simulink model "MyInverter_RTW"  (R2022a)
settings: Solver=ode1  StartTime=0.0  StopTime=inf  FixedStep=0.0002  RelTol=1e-3
PreLoadFcn:
  | vehicle = 'Car'; if ~length(which('cmself')), cmenv; end
  | MyInverter_RTW_bus
InitFcn:
  | vehicle = 'Car'; if ~length(which('cmself')), cmenv; end
  | MyInverter_RTW_bus
Description:
  | CarMaker Plug-in Model Target
settings Model: Creator=ml  LastModifiedBy=IPG
settings DebuggingCC: UnconnectedInputMsg=warning  UnconnectedOutputMsg=warning  UnconnectedLineMsg=warning
settings RTWCC: Description=CarMaker Plug-in Model Target  SystemTargetFile=CarMaker.tlc  TemplateMakefile=CarMaker_unix-win64.tmf  DLArmComputeVersion=19.05
settings CodeAppCC: MaxIdLength=127
settings STFCustomTargetCC: TargetLangStandard=C99 (ISO)  CombineOutputUpdateFcns=on  MatFileLogging=on  CodeInterfacePackaging=Reusable function  GRTInterface=off  GenerateAllocFcn=on  SystemTargetFile=CarMaker.tlc
settings GRTTargetCC: ParMdlRefBuildCompliant=off  CompOptLevelCompliant=off  ConcurrentExecutionCompliant=off  CodeInterfacePackaging=Reusable function  CPPClassGenCompliant=off  GenerateAllocFcn=on  UseToolchainInfoCompliant=off

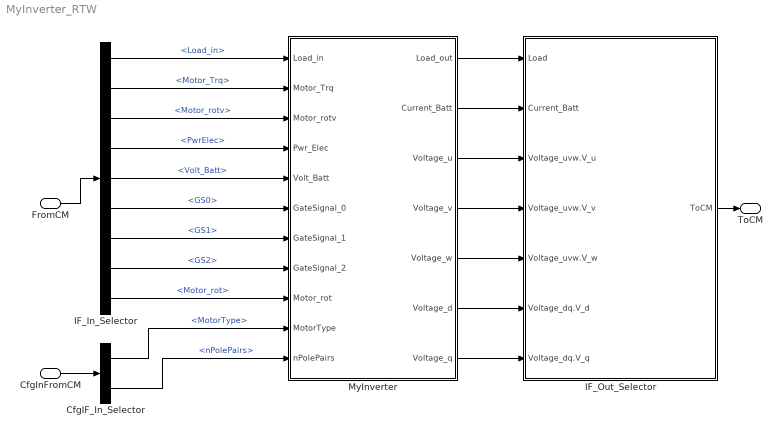
== system MyInverter_RTW ==
  FromCM : Inport  OutDataTypeStr=Bus: cmPTInverterIn
  CfgInFromCM : Inport  Port=2  OutDataTypeStr=Bus: cmPTInverterCfgIn
  CfgIF_In_Selector : BusSelector  OutputSignals=MotorType,nPolePairs
  IF_In_Selector : BusSelector  OutputSignals=Load_in,Motor_Trq,Motor_rotv,PwrElec,Volt_Batt,GateSignal.GS0,GateSignal.GS1,GateSignal.GS2,Motor_rot
  IF_Out_Selector : Subsystem  mask(Signal Selection){}
      mask help: Signal Selection Block
      settings: OpenFcn=cmSignalSelect('SignalSelection_CB',gcb)
  MyInverter : Subsystem
  ToCM : Outport  OutDataTypeStr=Bus: cmPTInverterOut
  wires:
  FromCM/1 -> IF_In_Selector/1
  IF_Out_Selector/1(ToCM) -> ToCM/1
  CfgInFromCM/1 -> CfgIF_In_Selector/1
  MyInverter/6(Voltage_d) -> IF_Out_Selector/6(Voltage_dq.V_d)
  IF_In_Selector/4 -> MyInverter/4(Pwr_Elec)  "<PwrElec>"
  IF_In_Selector/6 -> MyInverter/6(GateSignal_0)  "<GS0>"
  MyInverter/1(Load_out) -> IF_Out_Selector/1(Load)
  IF_In_Selector/9 -> MyInverter/9(Motor_rot)  "<Motor_rot>"
  IF_In_Selector/3 -> MyInverter/3(Motor_rotv)  "<Motor_rotv>"
  IF_In_Selector/2 -> MyInverter/2(Motor_Trq)  "<Motor_Trq>"
  MyInverter/5(Voltage_w) -> IF_Out_Selector/5(Voltage_uvw.V_w)
  CfgIF_In_Selector/2 -> MyInverter/11(nPolePairs)  "<nPolePairs>"
  IF_In_Selector/1 -> MyInverter/1(Load_in)  "<Load_in>"
  IF_In_Selector/7 -> MyInverter/7(GateSignal_1)  "<GS1>"
  MyInverter/3(Voltage_u) -> IF_Out_Selector/3(Voltage_uvw.V_u)
  IF_In_Selector/8 -> MyInverter/8(GateSignal_2)  "<GS2>"
  MyInverter/4(Voltage_v) -> IF_Out_Selector/4(Voltage_uvw.V_v)
  MyInverter/2(Current_Batt) -> IF_Out_Selector/2(Current_Batt)
  IF_In_Selector/5 -> MyInverter/5(Volt_Batt)  "<Volt_Batt>"
  MyInverter/7(Voltage_q) -> IF_Out_Selector/7(Voltage_dq.V_q)
  CfgIF_In_Selector/1 -> MyInverter/10(MotorType)  "<MotorType>"

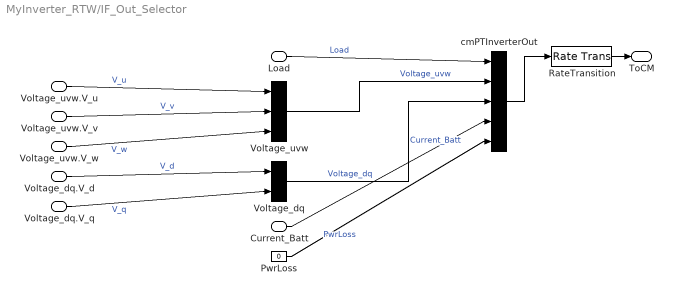
== system MyInverter_RTW/IF_Out_Selector ==
  Load : Inport
  Current_Batt : Inport  Port=2
  Voltage_uvw.V_u : Inport  Port=3
  Voltage_uvw.V_v : Inport  Port=4
  Voltage_uvw.V_w : Inport  Port=5
  Voltage_dq.V_d : Inport  Port=6
  Voltage_dq.V_q : Inport  Port=7
  PwrLoss : Constant  Value=0
  RateTransition : RateTransition  OutPortSampleTime=str2num(get_param(bdroot,'FixedStep'))
  Voltage_dq : BusCreator  Inputs=2
  Voltage_uvw : BusCreator  Inputs=3
  cmPTInverterOut : BusCreator  Inputs=5
  ToCM : Outport
  wires:
  RateTransition/1 -> ToCM/1
  cmPTInverterOut/1 -> RateTransition/1
  Voltage_uvw/1 -> cmPTInverterOut/2  "Voltage_uvw"
  Voltage_dq/1 -> cmPTInverterOut/3  "Voltage_dq"
  PwrLoss/1 -> cmPTInverterOut/5  "PwrLoss"
  Load/1 -> cmPTInverterOut/1  "Load"
  Current_Batt/1 -> cmPTInverterOut/4  "Current_Batt"
  Voltage_uvw.V_u/1 -> Voltage_uvw/1  "V_u"
  Voltage_uvw.V_v/1 -> Voltage_uvw/2  "V_v"
  Voltage_uvw.V_w/1 -> Voltage_uvw/3  "V_w"
  Voltage_dq.V_d/1 -> Voltage_dq/1  "V_d"
  Voltage_dq.V_q/1 -> Voltage_dq/2  "V_q"

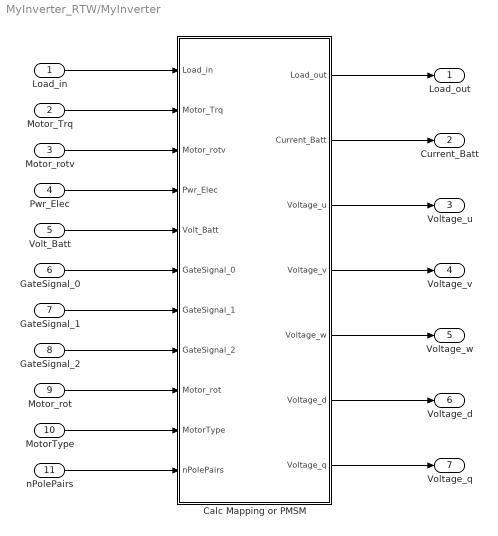
== system MyInverter_RTW/MyInverter ==
  Load_in : Inport
  Motor_Trq : Inport  Port=2
  Motor_rotv : Inport  Port=3
  Pwr_Elec : Inport  Port=4
  Volt_Batt : Inport  Port=5
  GateSignal_0 : Inport  Port=6
  GateSignal_1 : Inport  Port=7
  GateSignal_2 : Inport  Port=8
  Motor_rot : Inport  Port=9
  MotorType : Inport  Port=10
  nPolePairs : Inport  Port=11
  Calc Mapping or PMSM : Subsystem
  Load_out : Outport
  Current_Batt : Outport  Port=2
  Voltage_u : Outport  Port=3
  Voltage_v : Outport  Port=4
  Voltage_w : Outport  Port=5
  Voltage_d : Outport  Port=6
  Voltage_q : Outport  Port=7
  wires:
  Load_in/1 -> Calc Mapping or PMSM/1(Load_in)
  Motor_Trq/1 -> Calc Mapping or PMSM/2(Motor_Trq)
  Motor_rotv/1 -> Calc Mapping or PMSM/3(Motor_rotv)
  Pwr_Elec/1 -> Calc Mapping or PMSM/4(Pwr_Elec)
  Volt_Batt/1 -> Calc Mapping or PMSM/5(Volt_Batt)
  Calc Mapping or PMSM/1(Load_out) -> Load_out/1
  Calc Mapping or PMSM/2(Current_Batt) -> Current_Batt/1
  Calc Mapping or PMSM/3(Voltage_u) -> Voltage_u/1
  Calc Mapping or PMSM/4(Voltage_v) -> Voltage_v/1
  Calc Mapping or PMSM/5(Voltage_w) -> Voltage_w/1
  Calc Mapping or PMSM/6(Voltage_d) -> Voltage_d/1
  Calc Mapping or PMSM/7(Voltage_q) -> Voltage_q/1
  GateSignal_0/1 -> Calc Mapping or PMSM/6(GateSignal_0)
  GateSignal_1/1 -> Calc Mapping or PMSM/7(GateSignal_1)
  GateSignal_2/1 -> Calc Mapping or PMSM/8(GateSignal_2)
  MotorType/1 -> Calc Mapping or PMSM/10(MotorType)
  Motor_rot/1 -> Calc Mapping or PMSM/9(Motor_rot)
  nPolePairs/1 -> Calc Mapping or PMSM/11(nPolePairs)

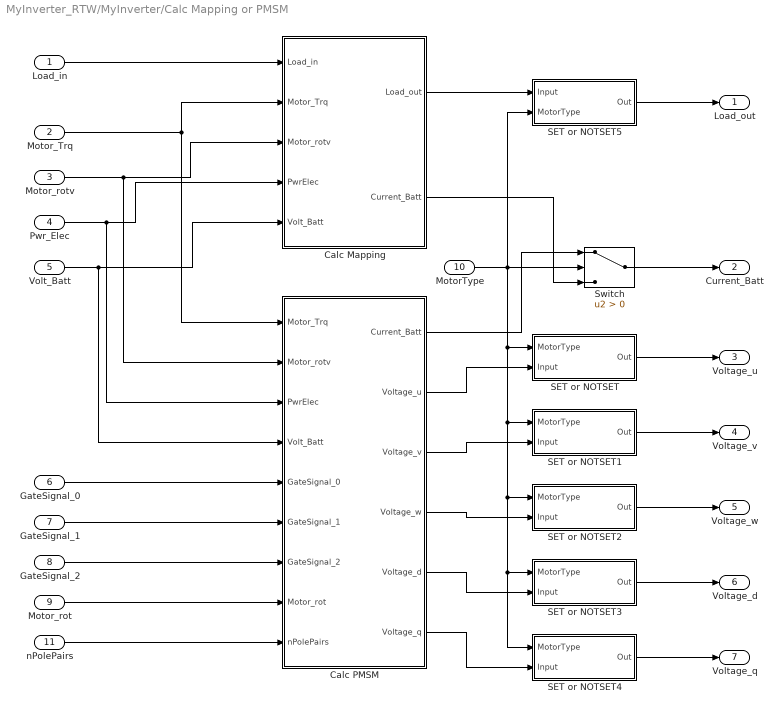
== system MyInverter_RTW/MyInverter/Calc Mapping or PMSM ==
  Load_in : Inport
  Motor_Trq : Inport  Port=2
  Motor_rotv : Inport  Port=3
  Pwr_Elec : Inport  Port=4
  Volt_Batt : Inport  Port=5
  GateSignal_0 : Inport  Port=6
  GateSignal_1 : Inport  Port=7
  GateSignal_2 : Inport  Port=8
  Motor_rot : Inport  Port=9
  MotorType : Inport  Port=10
  nPolePairs : Inport  Port=11
  Calc Mapping : Subsystem
  Calc PMSM : Subsystem
  SET or NOTSET : Subsystem
  SET or NOTSET1 : Subsystem
  SET or NOTSET2 : Subsystem
  SET or NOTSET3 : Subsystem
  SET or NOTSET4 : Subsystem
  SET or NOTSET5 : Subsystem
  Switch : Switch  Criteria=u2 > Threshold  SaturateOnIntegerOverflow=off  InputSameDT=off
  Load_out : Outport
  Current_Batt : Outport  Port=2
  Voltage_u : Outport  Port=3
  Voltage_v : Outport  Port=4
  Voltage_w : Outport  Port=5
  Voltage_d : Outport  Port=6
  Voltage_q : Outport  Port=7
  wires:
  Load_in/1 -> Calc Mapping/1(Load_in)
  Motor_Trq/1 -> Calc Mapping/2(Motor_Trq), Calc PMSM/1(Motor_Trq)
  Motor_rotv/1 -> Calc PMSM/2(Motor_rotv), Calc Mapping/3(Motor_rotv)
  Pwr_Elec/1 -> Calc PMSM/3(PwrElec), Calc Mapping/4(PwrElec)
  Volt_Batt/1 -> Calc PMSM/4(Volt_Batt), Calc Mapping/5(Volt_Batt)
  MotorType/1 -> SET or NOTSET5/2(MotorType), SET or NOTSET4/1(MotorType), SET or NOTSET3/1(MotorType), SET or NOTSET2/1(MotorType), SET or NOTSET1/1(MotorType), SET or NOTSET/1(MotorType), Switch/2
  Calc Mapping/2(Current_Batt) -> Switch/3
  Calc PMSM/1(Current_Batt) -> Switch/1
  Switch/1 -> Current_Batt/1
  Calc Mapping/1(Load_out) -> SET or NOTSET5/1(Input)
  GateSignal_0/1 -> Calc PMSM/5(GateSignal_0)
  GateSignal_1/1 -> Calc PMSM/6(GateSignal_1)
  GateSignal_2/1 -> Calc PMSM/7(GateSignal_2)
  Calc PMSM/2(Voltage_u) -> SET or NOTSET/2(Input)
  SET or NOTSET/1(Out) -> Voltage_u/1
  Calc PMSM/3(Voltage_v) -> SET or NOTSET1/2(Input)
  SET or NOTSET1/1(Out) -> Voltage_v/1
  Calc PMSM/4(Voltage_w) -> SET or NOTSET2/2(Input)
  SET or NOTSET2/1(Out) -> Voltage_w/1
  Calc PMSM/5(Voltage_d) -> SET or NOTSET3/2(Input)
  SET or NOTSET3/1(Out) -> Voltage_d/1
  Calc PMSM/6(Voltage_q) -> SET or NOTSET4/2(Input)
  SET or NOTSET4/1(Out) -> Voltage_q/1
  SET or NOTSET5/1(Out) -> Load_out/1
  Motor_rot/1 -> Calc PMSM/8(Motor_rot)
  nPolePairs/1 -> Calc PMSM/9(nPolePairs)

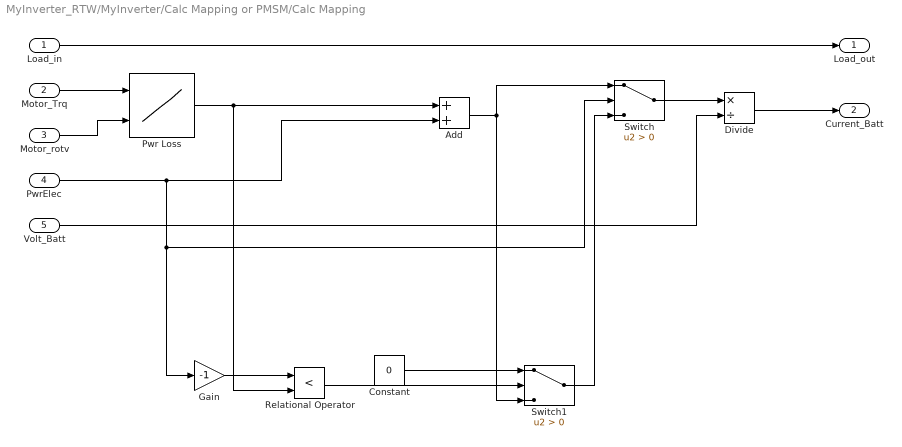
== system MyInverter_RTW/MyInverter/Calc Mapping or PMSM/Calc Mapping ==
  Load_in : Inport
  Motor_Trq : Inport  Port=2
  Motor_rotv : Inport  Port=3
  PwrElec : Inport  Port=4
  Volt_Batt : Inport  Port=5
  Add : Sum
  Constant : Constant  Value=0
  Divide : Product  Inputs=*/
  Gain : Gain  Gain=-1
  Pwr Loss : Lookup_n-D  BreakpointsForDimension1=[1,2,3]  BreakpointsForDimension2=[1,2,3]  Table=reshape([0,100,100,0,100,100,0,100,100],3,3)  InternalRulePriority=Speed  RndMeth=Simplest
      settings: InputPortMap=u0,u1
  Relational Operator : RelationalOperator  Operator=<  OutDataTypeStr=boolean  RndMeth=Simplest  InputSameDT=off
  Switch : Switch  Criteria=u2 > Threshold  SaturateOnIntegerOverflow=off  InputSameDT=off
  Switch1 : Switch  Criteria=u2 > Threshold  SaturateOnIntegerOverflow=off  InputSameDT=off
  Load_out : Outport
  Current_Batt : Outport  Port=2
  wires:
  Divide/1 -> Current_Batt/1
  Load_in/1 -> Load_out/1
  Switch1/1 -> Switch/3
  Gain/1 -> Relational Operator/1
  Motor_rotv/1 -> Pwr Loss/2
  Switch/1 -> Divide/1
  Pwr Loss/1 -> Relational Operator/2, Add/1
  Volt_Batt/1 -> Divide/2
  Motor_Trq/1 -> Pwr Loss/1
  Constant/1 -> Switch1/1
  Relational Operator/1 -> Switch1/2
  PwrElec/1 -> Gain/1, Switch/2, Add/2
  Add/1 -> Switch1/3, Switch/1

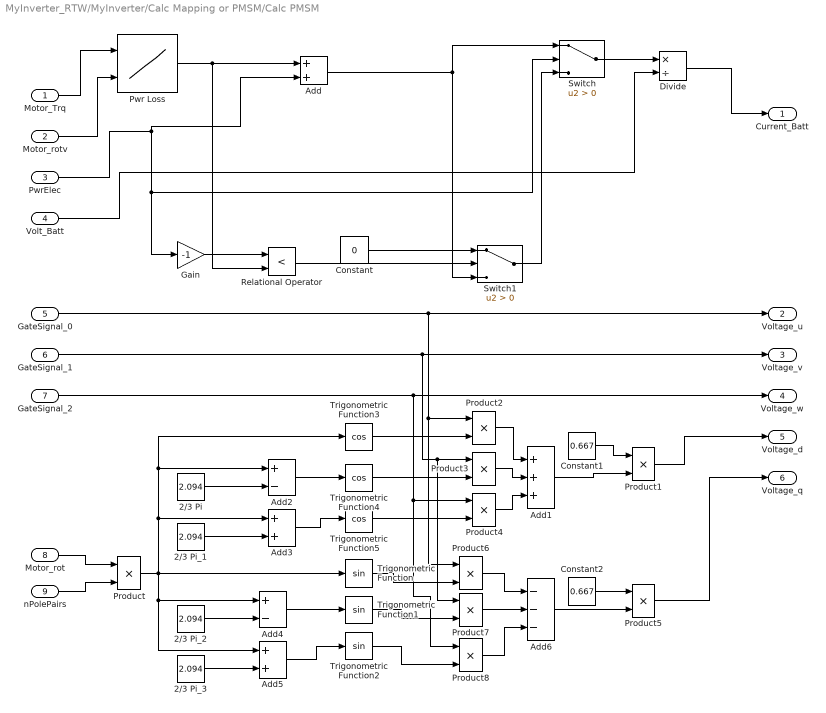
== system MyInverter_RTW/MyInverter/Calc Mapping or PMSM/Calc PMSM ==
  Motor_Trq : Inport
  Motor_rotv : Inport  Port=2
  PwrElec : Inport  Port=3
  Volt_Batt : Inport  Port=4
  GateSignal_0 : Inport  Port=5
  GateSignal_1 : Inport  Port=6
  GateSignal_2 : Inport  Port=7
  Motor_rot : Inport  Port=8
  nPolePairs : Inport  Port=9
  2/3 Pi : Constant  Value=2.094  OutDataTypeStr=double
  2/3 Pi_1 : Constant  Value=2.094  OutDataTypeStr=double
  2/3 Pi_2 : Constant  Value=2.094  OutDataTypeStr=double
  2/3 Pi_3 : Constant  Value=2.094  OutDataTypeStr=double
  Add : Sum
  Add1 : Sum  Inputs=+++
  Add2 : Sum  Inputs=+-
  Add3 : Sum
  Add4 : Sum  Inputs=+-
  Add5 : Sum
  Add6 : Sum  Inputs=---
  Constant : Constant  Value=0
  Constant1 : Constant  Value=0.667
  Constant2 : Constant  Value=0.667
  Divide : Product  Inputs=*/
  Gain : Gain  Gain=-1
  Product{,1..8} (9 alike) : Product
  Pwr Loss : Lookup_n-D  BreakpointsForDimension1=[1,2,3]  BreakpointsForDimension2=[1,2,3]  Table=reshape([0,100,100,0,100,100,0,100,100],3,3)  InternalRulePriority=Speed  RndMeth=Simplest
      settings: InputPortMap=u0,u1
  Relational Operator : RelationalOperator  Operator=<  OutDataTypeStr=boolean  RndMeth=Simplest  InputSameDT=off
  Switch : Switch  Criteria=u2 > Threshold  SaturateOnIntegerOverflow=off  InputSameDT=off
  Switch1 : Switch  Criteria=u2 > Threshold  SaturateOnIntegerOverflow=off  InputSameDT=off
  Trigonometric Function : Trigonometry  OutputSignalType=real
  Trigonometric Function1 : Trigonometry  OutputSignalType=real
  Trigonometric Function2 : Trigonometry  OutputSignalType=real
  Trigonometric Function3 : Trigonometry  Operator=cos  OutputSignalType=real
  Trigonometric Function4 : Trigonometry  Operator=cos  OutputSignalType=real
  Trigonometric Function5 : Trigonometry  Operator=cos  OutputSignalType=real
  Current_Batt : Outport
  Voltage_u : Outport  Port=2
  Voltage_v : Outport  Port=3
  Voltage_w : Outport  Port=4
  Voltage_d : Outport  Port=5
  Voltage_q : Outport  Port=6
  wires:
  Divide/1 -> Current_Batt/1
  Switch1/1 -> Switch/3
  Gain/1 -> Relational Operator/1
  Motor_rotv/1 -> Pwr Loss/2
  Switch/1 -> Divide/1
  Pwr Loss/1 -> Relational Operator/2, Add/1
  Volt_Batt/1 -> Divide/2
  Motor_Trq/1 -> Pwr Loss/1
  Constant/1 -> Switch1/1
  Relational Operator/1 -> Switch1/2
  PwrElec/1 -> Gain/1, Switch/2, Add/2
  Add/1 -> Switch1/3, Switch/1
  GateSignal_0/1 -> Product6/1, Product2/1, Voltage_u/1
  GateSignal_1/1 -> Product7/1, Product3/1, Voltage_v/1
  GateSignal_2/1 -> Product8/1, Product4/1, Voltage_w/1
  Motor_rot/1 -> Product/1
  nPolePairs/1 -> Product/2
  Add1/1 -> Product1/2
  Constant1/1 -> Product1/1
  Product1/1 -> Voltage_d/1
  2/3 Pi/1 -> Add2/2
  Add2/1 -> Trigonometric Function4/1
  2/3 Pi_1/1 -> Add3/2
  Add3/1 -> Trigonometric Function5/1
  Trigonometric Function3/1 -> Product2/2
  Product2/1 -> Add1/1
  Trigonometric Function4/1 -> Product3/2
  Product3/1 -> Add1/2
  Trigonometric Function5/1 -> Product4/2
  Product4/1 -> Add1/3
  Product/1 -> Trigonometric Function/1, Add3/1, Trigonometric Function3/1, Add2/1, Add5/1, Add4/1
  2/3 Pi_2/1 -> Add4/2
  Add4/1 -> Trigonometric Function1/1
  Add5/1 -> Trigonometric Function2/1
  2/3 Pi_3/1 -> Add5/2
  Constant2/1 -> Product5/1
  Add6/1 -> Product5/2
  Trigonometric Function/1 -> Product6/2
  Product6/1 -> Add6/1
  Trigonometric Function1/1 -> Product7/2
  Product7/1 -> Add6/2
  Trigonometric Function2/1 -> Product8/2
  Product8/1 -> Add6/3
  Product5/1 -> Voltage_q/1

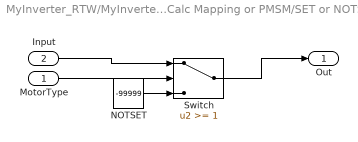
== system MyInverter_RTW/MyInverter/Calc Mapping or PMSM/SET or NOTSET ==
  MotorType : Inport
  Input : Inport  Port=2
  NOTSET : Constant  Value=-99999
  Switch : Switch  Threshold=1  SaturateOnIntegerOverflow=off  InputSameDT=off
  Out : Outport
  wires:
  MotorType/1 -> Switch/2
  Input/1 -> Switch/1
  NOTSET/1 -> Switch/3
  Switch/1 -> Out/1

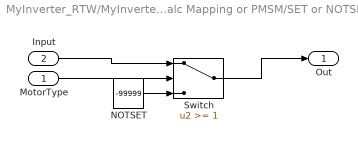
== system MyInverter_RTW/MyInverter/Calc Mapping or PMSM/SET or NOTSET1 ==
  MotorType : Inport
  Input : Inport  Port=2
  NOTSET : Constant  Value=-99999
  Switch : Switch  Threshold=1  SaturateOnIntegerOverflow=off  InputSameDT=off
  Out : Outport
  wires:
  MotorType/1 -> Switch/2
  Input/1 -> Switch/1
  NOTSET/1 -> Switch/3
  Switch/1 -> Out/1

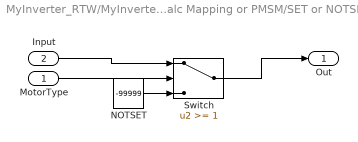
== system MyInverter_RTW/MyInverter/Calc Mapping or PMSM/SET or NOTSET2 ==
  MotorType : Inport
  Input : Inport  Port=2
  NOTSET : Constant  Value=-99999
  Switch : Switch  Threshold=1  SaturateOnIntegerOverflow=off  InputSameDT=off
  Out : Outport
  wires:
  MotorType/1 -> Switch/2
  Input/1 -> Switch/1
  NOTSET/1 -> Switch/3
  Switch/1 -> Out/1

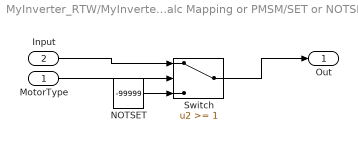
== system MyInverter_RTW/MyInverter/Calc Mapping or PMSM/SET or NOTSET3 ==
  MotorType : Inport
  Input : Inport  Port=2
  NOTSET : Constant  Value=-99999
  Switch : Switch  Threshold=1  SaturateOnIntegerOverflow=off  InputSameDT=off
  Out : Outport
  wires:
  MotorType/1 -> Switch/2
  Input/1 -> Switch/1
  NOTSET/1 -> Switch/3
  Switch/1 -> Out/1

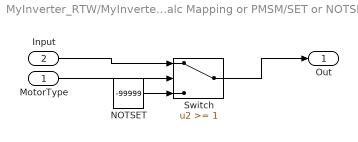
== system MyInverter_RTW/MyInverter/Calc Mapping or PMSM/SET or NOTSET4 ==
  MotorType : Inport
  Input : Inport  Port=2
  NOTSET : Constant  Value=-99999
  Switch : Switch  Threshold=1  SaturateOnIntegerOverflow=off  InputSameDT=off
  Out : Outport
  wires:
  MotorType/1 -> Switch/2
  Input/1 -> Switch/1
  NOTSET/1 -> Switch/3
  Switch/1 -> Out/1

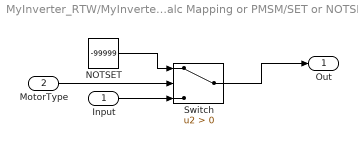
== system MyInverter_RTW/MyInverter/Calc Mapping or PMSM/SET or NOTSET5 ==
  Input : Inport
  MotorType : Inport  Port=2
  NOTSET : Constant  Value=-99999
  Switch : Switch  Criteria=u2 > Threshold  SaturateOnIntegerOverflow=off  InputSameDT=off
  Out : Outport
  wires:
  MotorType/1 -> Switch/2
  Input/1 -> Switch/3
  NOTSET/1 -> Switch/1
  Switch/1 -> Out/1
